simulink model "Zad_4_sch"  (R2022a)
settings: Solver=VariableStepAuto  StartTime=0.0  StopTime=10.0  RelTol=1e-3
values from neighbouring files (symbols this model uses):
  a21 = (1/(2*m))*x30^2*(FemP1/FemP2^2)*exp(-x10/FemP2)    [Zad_2.m]
  a23 = -(1/m)*x30*(FemP1/FemP2)*exp(-x10/FemP2)    [Zad_2.m]
  a31 = (1/f1)*exp(x10/f2)*(ki*u10+ci-x30)    [Zad_2.m]
  a33 = -(f2/f1)*exp(x10/f2)    [Zad_2.m]
  b31 = ki*(f2/f1)*exp(x10/f2)    [Zad_2.m]
  g = 9.81    [Zad_2.m]
  K1 = 1    [Zad_4.m]
  K2 = 1    [Zad_4.m]
  K3ddyr = 1/a23    [Zad_4.m]
  K3g = -1/a23    [Zad_4.m]
  K3yr = -a21/a23    [Zad_4.m]
  Kdddyr = 1/(b31*a23)    [Zad_4.m]
  Kddyr = -(a33)/(a23*b31)    [Zad_4.m]
  Kdyr = -(a21)/(a23*b31)    [Zad_4.m]
  Kg = a33/(a23*b31)    [Zad_4.m]
  Kxpom = place(A,Bpom,p_d)    [Zad_4.m]    (also in Zad_5.m; Zad_6.m)
  Kyr = (a21*a33-a31*a23)/(a23*b31)    [Zad_4.m]
  xd = d-bd    (= 0.01326)    [Zad_2.m]
settings Model: Creator=marci  LastModifiedBy=marci
settings SolverCC: ZeroCrossAlgorithm=Adaptive
settings DebuggingCC: IgnoredZcDiagnostic=none

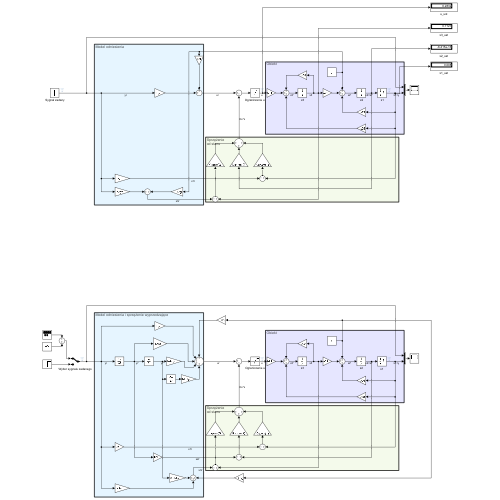
[thumbnail: Simulink's stored preview of the top-level diagram]
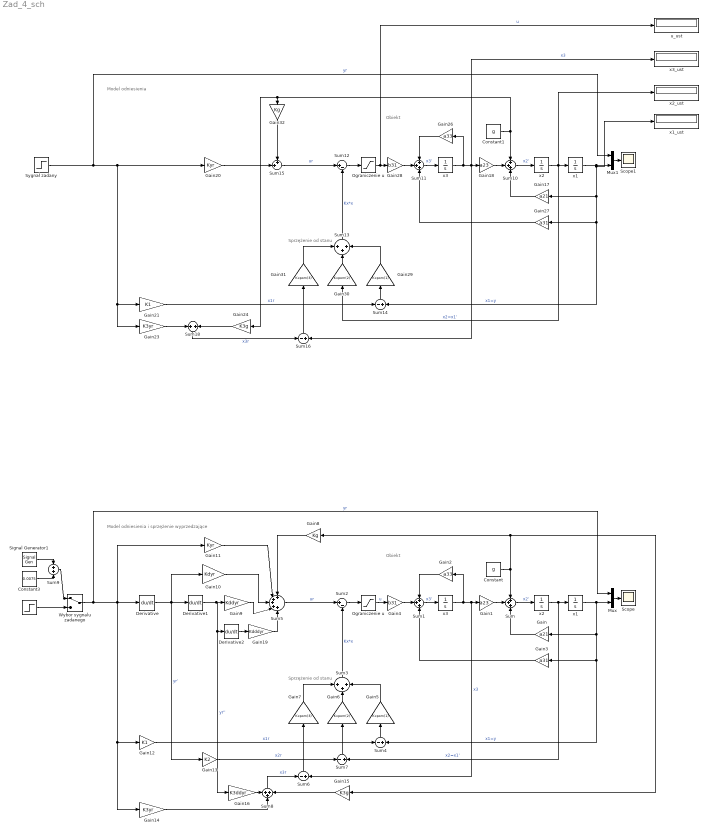
== system Zad_4_sch ==
  note: Sprzężenie
      | od stanu
  note: Model odniesienia i sprzężenie wyprzedzające
  note: Obiekt
  note: Sprzężenie
      | od stanu
  note: Model odniesienia
  note: Obiekt
  "  " : Step  Time=0  After=0.008  SampleTime=0
  " Sygnał zadany" : Step  Time=0  After=0.008  SampleTime=0
  " x1" : Integrator  InitialCondition=xd  LimitOutput=on  UpperSaturationLimit=xd  LowerSaturationLimit=0
  " x2" : Integrator
  " x3" : Integrator
  Constant : Constant  Value=g
  Constant1 : Constant  Value=g
  Constant3 : Constant  Value=0.0075
  Derivative : Derivative
  Derivative1 : Derivative
  Derivative2 : Derivative
  Gain : Gain  Gain=a21
  Gain1 : Gain  Gain=a23
  Gain10 : Gain  Gain=Kdyr
  Gain11 : Gain  Gain=Kyr
  Gain12 : Gain  Gain=K1
  Gain13 : Gain  Gain=K2
  Gain14 : Gain  Gain=K3yr
  Gain15 : Gain  Gain=K3g
  Gain16 : Gain  Gain=K3ddyr
  Gain17 : Gain  Gain=a21
  Gain18 : Gain  Gain=a23
  Gain19 : Gain  Gain=Kdddyr
  Gain2 : Gain  Gain=a33
  Gain20 : Gain  Gain=Kyr
  Gain21 : Gain  Gain=K1
  Gain23 : Gain  Gain=K3yr
  Gain24 : Gain  Gain=K3g
  Gain26 : Gain  Gain=a33
  Gain27 : Gain  Gain=a31
  Gain28 : Gain  Gain=b31
  Gain29 : Gain  Gain=Kxpom(1)
  Gain3 : Gain  Gain=a31
  Gain30 : Gain  Gain=Kxpom(2)
  Gain31 : Gain  Gain=Kxpom(3)
  Gain32 : Gain  Gain=Kg
  Gain4 : Gain  Gain=b31
  Gain5 : Gain  Gain=Kxpom(1)
  Gain6 : Gain  Gain=Kxpom(2)
  Gain7 : Gain  Gain=Kxpom(3)
  Gain8 : Gain  Gain=Kg
  Gain9 : Gain  Gain=Kddyr
  Mux : Mux  Inputs=2
  Mux1 : Mux  Inputs=2
  Ograniczenie u : Saturate  UpperLimit=1  LowerLimit=0  ZeroCross=off
  "Ograniczenie u " : Saturate  UpperLimit=1  LowerLimit=0  ZeroCross=off
  Scope : Scope
  Scope1 : Scope
  Signal Generator1 : SignalGenerator  Amplitude=0.005  Frequency=4  Units=rad/sec
  Sum{,1,3,8,10..11,13} (7 alike) : Sum  Inputs=+++
  Sum12 : Sum  Inputs=|+-
  Sum{4,6..7,14,16} (5 alike) : Sum  Inputs=-+
  Sum15 : Sum  Inputs=++|
  Sum18 : Sum
  Sum2 : Sum  Inputs=|+-
  Sum5 : Sum  Inputs=+++++
  Sum9 : Sum
  Wybor sygnalu zadanego : ManualSwitch
  u_ust : Display
  x1 : Integrator  InitialCondition=xd  LimitOutput=on  UpperSaturationLimit=xd  LowerSaturationLimit=0
  x1_ust : Display
  x2 : Integrator
  x2_ust : Display
  x3 : Integrator
  x3_ust : Display
  wires:
  Gain2/1 -> Sum1/1
  Sum1/1 -> x3/1  "x3'"
  Gain1/1 -> Sum/2
  Gain4/1 -> Sum1/2
  Sum/1 -> x2/1  "x2'"
  Gain3/1 -> Sum1/3
  Constant/1 -> Sum/1, Gain8/1, Gain15/1
  Sum2/1 -> Ograniczenie u/1
  Gain/1 -> Sum/3
  Sum3/1 -> Sum2/2  "Kx*x"
  Sum6/1 -> Gain7/1
  Gain5/1 -> Sum3/3
  Gain6/1 -> Sum3/2
  Gain7/1 -> Sum3/1
  Sum4/1 -> Gain5/1
  Wybor sygnalu zadanego/1 -> Mux/1, Gain14/1, Gain12/1, Gain11/1, Derivative/1  "yr"
  Derivative/1 -> Gain13/1, Gain10/1, Derivative1/1  "yr'"
  Sum5/1 -> Sum2/1  "ur"
  Gain8/1 -> Sum5/1
  Derivative1/1 -> Derivative2/1, Gain16/1, Gain9/1  "yr''"
  Sum7/1 -> Gain6/1
  Gain9/1 -> Sum5/4
  Gain10/1 -> Sum5/3
  Gain11/1 -> Sum5/2
  Gain12/1 -> Sum4/1  "x1r"
  Gain13/1 -> Sum7/1  "x2r"
  Sum8/1 -> Sum6/1  "x3r"
  Gain15/1 -> Sum8/3
  Gain16/1 -> Sum8/1
  Gain14/1 -> Sum8/2
  Signal Generator1/1 -> Sum9/1
  "  "/1 -> Wybor sygnalu zadanego/2
  Constant3/1 -> Sum9/2
  Sum9/1 -> Wybor sygnalu zadanego/1
  Mux/1 -> Scope/1
  Gain23/1 -> Sum18/1
  Gain31/1 -> Sum13/1
  Gain28/1 -> Sum11/2
  " x2"/1 -> x2_ust/1, Gain30/1, " x1"/1  "x2=x1'"
  Gain21/1 -> Sum14/1  "x1r"
  " x1"/1 -> Mux1/2, x1_ust/1, Gain17/1, Sum14/2, Gain27/1  "x1=y"
  "Ograniczenie u "/1 -> u_ust/1, Gain28/1  "u"
  Sum15/1 -> Sum12/1  "ur"
  Gain24/1 -> Sum18/2
  Gain18/1 -> Sum10/2
  Gain20/1 -> Sum15/2
  Sum13/1 -> Sum12/2  "Kx*x"
  Sum14/1 -> Gain29/1
  Gain32/1 -> Sum15/1
  Gain30/1 -> Sum13/2
  Gain29/1 -> Sum13/3
  " Sygnał zadany"/1 -> Mux1/1, Gain20/1, Gain23/1, Gain21/1  "yr"
  Gain26/1 -> Sum11/1
  Mux1/1 -> Scope1/1
  Sum16/1 -> Gain31/1
  Sum12/1 -> "Ograniczenie u "/1
  Constant1/1 -> Sum10/1, Gain32/1, Gain24/1
  Gain17/1 -> Sum10/3
  Sum18/1 -> Sum16/1  "x3r"
  Gain27/1 -> Sum11/3
  " x3"/1 -> x3_ust/1, Sum16/2, Gain18/1, Gain26/1  "x3"
  Sum11/1 -> " x3"/1  "x3'"
  Sum10/1 -> " x2"/1  "x2'"
  Derivative2/1 -> Gain19/1
  Gain19/1 -> Sum5/5
  x2/1 -> Sum7/2, x1/1  "x2=x1'"
  x1/1 -> Mux/2, Gain/1, Sum4/2, Gain3/1  "x1=y"
  Ograniczenie u/1 -> Gain4/1  "u"
  x3/1 -> Gain2/1, Sum6/2, Gain1/1  "x3"
